simulink model "doubleIntegrator"  (R2018a)
settings: Solver=FixedStepAuto  StartTime=0.0  StopTime=2.0  FixedStep=0.001  RelTol=1e-9  AbsTol=1e-12
settings Model: Creator=george  LastModifiedBy=george
settings CodeAppCC: StateflowObjectComments=on

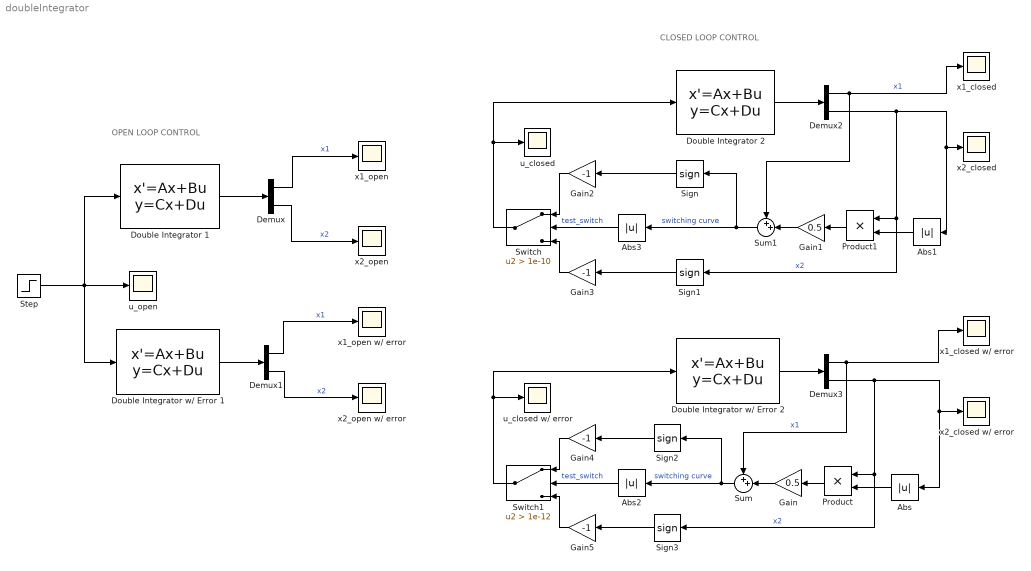
== system doubleIntegrator ==
  note: CLOSED LOOP CONTROL
  note: OPEN LOOP CONTROL
  Abs{,1..3} (4 alike) : Abs
  Demux{,1..3} (4 alike) : Demux  Outputs=2
  Double Integrator w/ Error 1 : StateSpace  A=[0 1; 0 0]  B=[0; 1.1]  C=[1 0; 0 1]  D=[0; 0]  InitialCondition=[-1; 0]
  Double Integrator w/ Error 2 : StateSpace  A=[0 1; 0 0]  B=[0; 1.1]  C=[1 0; 0 1]  D=[0; 0]  InitialCondition=[-1; 0]
  Double Integrator 1 : StateSpace  A=[0 1; 0 0]  B=[0; 1]  C=[1 0; 0 1]  D=[0; 0]  InitialCondition=[-1; 0]
  Double Integrator 2 : StateSpace  A=[0 1; 0 0]  B=[0; 1]  C=[1 0; 0 1]  D=[0; 0]  InitialCondition=[-1; 0]
  Gain : Gain  Gain=0.5
  Gain1 : Gain  Gain=0.5
  Gain{2..5} (4 alike) : Gain  Gain=-1
  Product : Product
  Product1 : Product
  Sign{,1..3} (4 alike) : Signum
  Step : Step  Before=1  After=-1  SampleTime=0
  Sum : Sum  Inputs=++|
  Sum1 : Sum  Inputs=++|
  Switch : Switch  Criteria=u2 > Threshold  Threshold=1e-10
  Switch1 : Switch  Criteria=u2 > Threshold  Threshold=1e-12
  u_closed : Scope
  u_closed w/ error : Scope
  u_open : Scope
  x1_closed : Scope
  x1_closed w/ error : Scope
  x1_open : Scope
  x1_open w/ error : Scope
  x2_closed : Scope
  x2_closed w/ error : Scope
  x2_open : Scope
  x2_open w/ error : Scope
  wires:
  Demux3/1 -> x1_closed w/ error/1, Sum/1  "x1"
  Double Integrator w/ Error 2/1 -> Demux3/1
  Demux3/2 -> Abs/1, x2_closed w/ error/1, Sign3/1, Product/1  "x2"
  Double Integrator 2/1 -> Demux2/1
  Demux2/2 -> Sign1/1, Product1/1, x2_closed/1, Abs1/1  "x2"
  Demux2/1 -> Sum1/1, x1_closed/1  "x1"
  Gain/1 -> Sum/2
  Product/1 -> Gain/1
  Abs/1 -> Product/2
  Product1/1 -> Gain1/1
  Gain1/1 -> Sum1/2
  Abs1/1 -> Product1/2
  Sum1/1 -> Sign/1, Abs3/1  "switching curve"
  Sum/1 -> Sign2/1, Abs2/1  "switching curve"
  Sign/1 -> Gain2/1
  Gain2/1 -> Switch/1
  Sign1/1 -> Gain3/1
  Gain3/1 -> Switch/3
  Switch/1 -> u_closed/1, Double Integrator 2/1
  Gain4/1 -> Switch1/1
  Sign2/1 -> Gain4/1
  Sign3/1 -> Gain5/1
  Gain5/1 -> Switch1/3
  Switch1/1 -> Double Integrator w/ Error 2/1, u_closed w/ error/1
  Demux1/2 -> x2_open w/ error/1  "x2"
  Demux/2 -> x2_open/1  "x2"
  Step/1 -> u_open/1, Double Integrator w/ Error 1/1, Double Integrator 1/1
  Demux1/1 -> x1_open w/ error/1  "x1"
  Double Integrator w/ Error 1/1 -> Demux1/1
  Demux/1 -> x1_open/1  "x1"
  Double Integrator 1/1 -> Demux/1
  Abs2/1 -> Switch1/2  "test_switch"
  Abs3/1 -> Switch/2  "test_switch"
